simulink model "MultiSizeCells_IaF"  (R2020b)
settings: Solver=VariableStepAuto  StartTime=0.0  StopTime=2.0  RelTol=1e-3
libraries: NeuroModelerLibrary x10
settings Model: Creator=Александра  LastModifiedBy=Александра

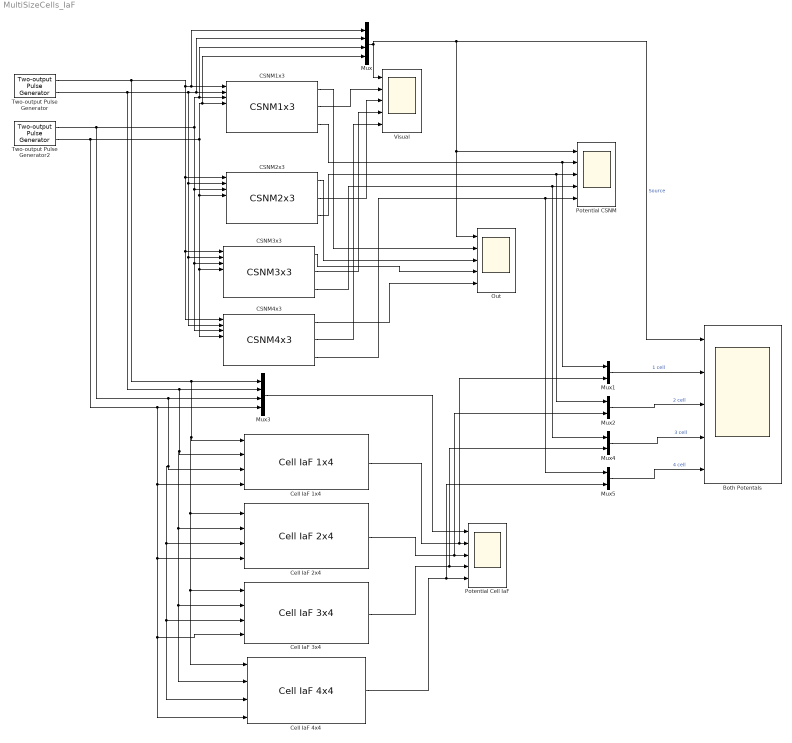
== system MultiSizeCells_IaF ==
  Both Potentals : Scope  NumInputPorts=5
  CSNM1x3 : NeuroModelerLibrary/Sized Cells/CSNM1x3  SystemSampleTime=-1  VariantActivationTime=update diagram  Latency=0  AutoFrameSizeCalculation=off
  CSNM2x3 : NeuroModelerLibrary/Sized Cells/CSNM2x3  SystemSampleTime=-1  VariantActivationTime=update diagram  Latency=0  AutoFrameSizeCalculation=off
  CSNM3x3 : NeuroModelerLibrary/Sized Cells/CSNM3x3  SystemSampleTime=-1  VariantActivationTime=update diagram  Latency=0  AutoFrameSizeCalculation=off
  CSNM4x3 : NeuroModelerLibrary/Sized Cells/CSNM4x3  SystemSampleTime=-1  VariantActivationTime=update diagram  Latency=0  AutoFrameSizeCalculation=off
  Cell IaF 1x4 : NeuroModelerLibrary/Sized Cells/Cell IaF 1x4  SystemSampleTime=-1  VariantActivationTime=update diagram  Latency=0  AutoFrameSizeCalculation=off
  Cell IaF 2x4 : NeuroModelerLibrary/Sized Cells/Cell IaF 2x4  SystemSampleTime=-1  VariantActivationTime=update diagram  Latency=0  AutoFrameSizeCalculation=off
  Cell IaF 3x4 : NeuroModelerLibrary/Sized Cells/Cell IaF 3x4  SystemSampleTime=-1  VariantActivationTime=update diagram  Latency=0  AutoFrameSizeCalculation=off
  Cell IaF 4x4 : NeuroModelerLibrary/Sized Cells/Cell IaF 4x4  SystemSampleTime=-1  VariantActivationTime=update diagram  Latency=0  AutoFrameSizeCalculation=off
  Mux : Mux
  Mux{1..2,4..5} (4 alike) : Mux  Inputs=2
  Mux3 : Mux
  Out : Scope  NumInputPorts=5
  Potential CSNM : Scope  NumInputPorts=5
  Potential Cell IaF : Scope  NumInputPorts=5
  Two-output Pulse Generator : NeuroModelerLibrary/Support/Two-output Pulse Generator  A=1  P1=200  P2=200  PW=1  ST=0.001  OOn1=0.5  OOff1=0.6  OOn2=0.8  OOff2=0.9
  Two-output Pulse Generator2 : NeuroModelerLibrary/Support/Two-output Pulse Generator  A=1  P1=200  P2=200  PW=1  ST=0.001  OOn1=1.2  OOff1=1.3  OOn2=1.6  OOff2=1.7
  Visual : Scope  NumInputPorts=5
  wires:
  Mux3/1 -> Potential Cell IaF/1
  CSNM1x3/2 -> Visual/2
  CSNM3x3/1 -> Out/4
  Two-output Pulse Generator/2 -> Cell IaF 1x4/2, Cell IaF 2x4/2, Cell IaF 4x4/2, Cell IaF 3x4/2, Mux3/2, CSNM1x3/2, Mux/2, CSNM2x3/2, CSNM4x3/2, CSNM3x3/2
  Two-output Pulse Generator2/2 -> Cell IaF 1x4/4, Cell IaF 2x4/4, Cell IaF 4x4/4, Cell IaF 3x4/4, Mux3/4, CSNM1x3/4, Mux/4, CSNM2x3/4, CSNM4x3/4, CSNM3x3/4
  CSNM4x3/1 -> Out/5
  Two-output Pulse Generator/1 -> Mux3/1, Cell IaF 1x4/1, Cell IaF 2x4/1, Cell IaF 4x4/1, Cell IaF 3x4/1, CSNM1x3/1, Mux/1, CSNM2x3/1, CSNM4x3/1, CSNM3x3/1
  CSNM3x3/3 -> Mux4/1, Potential CSNM/4
  CSNM2x3/2 -> Visual/3
  CSNM4x3/2 -> Visual/5
  Two-output Pulse Generator2/1 -> CSNM1x3/3, Mux/3, CSNM2x3/3, CSNM4x3/3, CSNM3x3/3, Cell IaF 1x4/3, Cell IaF 2x4/3, Cell IaF 4x4/3, Cell IaF 3x4/3, Mux3/3
  CSNM4x3/3 -> Mux5/1, Potential CSNM/5
  CSNM3x3/2 -> Visual/4
  CSNM2x3/1 -> Out/3
  CSNM1x3/1 -> Out/2
  CSNM2x3/3 -> Mux2/1, Potential CSNM/3
  CSNM1x3/3 -> Mux1/1, Potential CSNM/2
  Cell IaF 1x4/1 -> Mux1/2, Potential Cell IaF/2
  Cell IaF 2x4/1 -> Mux2/2, Potential Cell IaF/3
  Cell IaF 3x4/1 -> Mux4/2, Potential Cell IaF/4
  Cell IaF 4x4/1 -> Mux5/2, Potential Cell IaF/5
  Mux1/1 -> Both Potentals/2  "1 cell"
  Mux2/1 -> Both Potentals/3  "2 cell"
  Mux4/1 -> Both Potentals/4  "3 cell"
  Mux5/1 -> Both Potentals/5  "4 cell"
  Mux/1 -> Both Potentals/1, Out/1, Potential CSNM/1, Visual/1  "Source"
